simulink model "prj_autom"  (R2020b)
settings: Solver=VariableStepAuto  StartTime=0.0  StopTime=24.0  RelTol=1e-3
libraries: simulink x2
settings Model: Creator=xoxox  LastModifiedBy=xoxox

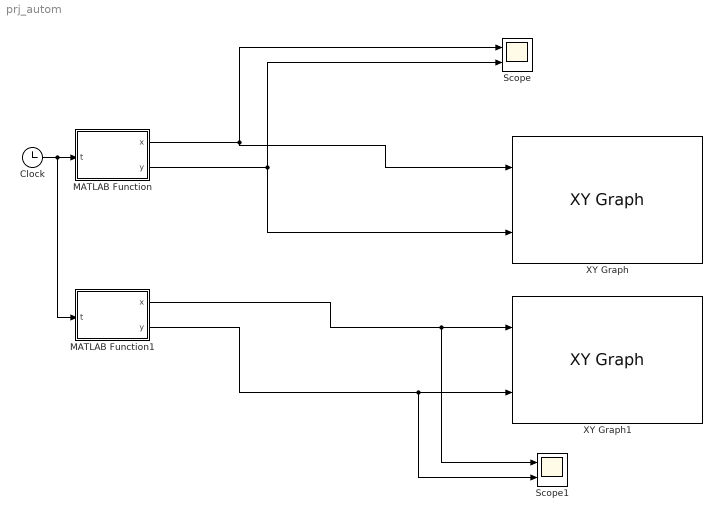
== system prj_autom ==
  Clock : Clock
  MATLAB Function : MATLAB Function  TreatAsAtomicUnit=on
  MATLAB Function1 : MATLAB Function  TreatAsAtomicUnit=on
  Scope : Scope  NumInputPorts=2
  Scope1 : Scope  NumInputPorts=2
  XY Graph : simulink/Sinks/XY Graph  xmin=-4  xmax=4  ymin=-4  ymax=4  st=-1
  XY Graph1 : simulink/Sinks/XY Graph  xmin=-10  xmax=10  ymin=-10  ymax=10  st=-1
  wires:
  Clock/1 -> MATLAB Function1/1(t), MATLAB Function/1(t)
  MATLAB Function/2(y) -> XY Graph/2, Scope/2
  MATLAB Function/1(x) -> XY Graph/1, Scope/1
  MATLAB Function1/1(x) -> Scope1/1, XY Graph1/1
  MATLAB Function1/2(y) -> Scope1/2, XY Graph1/2

== matlab function prj_autom/MATLAB Function ==
  data: t input; x output; y output
function [x,y] = fcn(t)
    TIME_BASE = 6;
    tt = mod(t,TIME_BASE);
    
    if(tt < TIME_BASE*2/6)
        x = 0;
        y = tt;
    else
        if(tt < TIME_BASE*3/6)
            x = sin((tt-TIME_BASE*2/6)*pi/2);
            y = sin((tt-TIME_BASE*2/6)*pi/2)+TIME_BASE*2/6;
        else
            if(tt < TIME_BASE*5/6)
                x = 1;
                y = -(tt-TIME_BASE*3/6)+TIME_BASE*3/6;
            else
                x = -sin((tt-TIME_BASE*5/6)*pi/2)+1;
                y = -sin((tt-TIME_BASE*5/6)*pi/2)+1;
            end
        end
    end
end

== matlab function prj_autom/MATLAB Function1 ==
  data: t input; x output; y output
function [x,y] = fcn(t)
    TIME_BASE = 12;
    tt = mod(t,TIME_BASE);
    
    if(tt < 4)
        x = 0;
        y = tt;
    else
        if(tt < 5)
            x = (tt-4)^2;
            y = sqrt(tt-4)+4;
            %y = (tt-4)^2+4;
        else
            if(tt < 6)
                x = sqrt(tt-5)+1;
                y = -(tt-5)^2+5;
                %y = -sqrt(tt-5)+5;
            else
                if(tt < 10)
                    x = 2;
                    y = -(tt-6)+4;
                else
                    if(tt < 11)
                        x = -(tt-10)^2+2;
                        y = -sqrt(tt-10);
                    else
                        x = -sqrt(tt-11)+1;
                        y = (tt-11)^2-1;
                    end
                end
            end
        end
    end
end
